simulink model "PassiveHydPTO"  (R2014a)
settings: Solver=ode23tb  StartTime=0.0  StopTime=param.stop  FixedStep=0.01  MaxStep=0.05  RelTol=1e-6
values from neighbouring files (symbols this model uses):
  alpha = 1    [passive_hydraulic_PTO.m]
  Amax = 0.001    [passive_hydraulic_PTO.m]
  Amin = 1e-8    (= 1e-08)    [passive_hydraulic_PTO.m]
  Ap = 2.35e-2    (= 0.0235)    [passive_hydraulic_PTO.m]
  Beta_e = 1.86e9    (= 1860000000)    [passive_hydraulic_PTO.m]
  bf = 0.05*bg    (= 0.118735)    [passive_hydraulic_PTO.m]
  bg = 2.3747    [passive_hydraulic_PTO.m]
  Cd = 0.61    [passive_hydraulic_PTO.m]
  D = 3.9789e-5    (= 3.9789e-05)    [passive_hydraulic_PTO.m]
  Dh = sqrt(4*Av/pi)    [passive_hydraulic_PTO.m]
  f = 1/period    (= 0.1)    [passive_hydraulic_PTO.m]
  J = 3.961    [passive_hydraulic_PTO.m]
  k1 = 200    [passive_hydraulic_PTO.m]
  k2 = atanh((Amin-(Amax-Amin)/2)*      2/(Amax - Amin))*1/(pMin-(pMax + pMin)/2)    [passive_hydraulic_PTO.m]
  omega_i = 0    [passive_hydraulic_PTO.m]
  pAeq = pCeq    (= 21333333.3333)    [passive_hydraulic_PTO.m]
  pAi = pAeq    (= 21333333.3333)    [passive_hydraulic_PTO.m]
  pAupper_limit = 32e6    (= 32000000)    [passive_hydraulic_PTO.m]
  pBeq = pCeq    (= 21333333.3333)    [passive_hydraulic_PTO.m]
  pBi = pBeq    (= 21333333.3333)    [passive_hydraulic_PTO.m]
  pBupper_limit = 32e6    (= 32000000)    [passive_hydraulic_PTO.m]
  pCprecharge = 0.9*pClower_limit    (= 19200000)    [passive_hydraulic_PTO.m]
  pDprecharge = 0.9*pDlower_limit    (= 9600000)    [passive_hydraulic_PTO.m]
  pMax = 1e6    (= 1000000)    [passive_hydraulic_PTO.m]
  pMin = 0.75e6    (= 750000)    [passive_hydraulic_PTO.m]
  rho = 850    [passive_hydraulic_PTO.m]
  Rt = 10    [passive_hydraulic_PTO.m]
  v = 5.5e-5    (= 5.5e-05)    [passive_hydraulic_PTO.m]
  VC0 = 7.5    [passive_hydraulic_PTO.m]
  VCeq = VC0*(1-(pCprecharge/pCeq)^(1/1.4))    (= 0.543715404282)    [passive_hydraulic_PTO.m]
  VD0 = 3    [passive_hydraulic_PTO.m]
  VDeq = VDmax    (= 1.30403881906)    [passive_hydraulic_PTO.m]
  Vo = Ap*5    (= 0.1175)    [passive_hydraulic_PTO.m]
undefined symbols (not defined in the file or in its folder): magnitude
settings Model: Creator=sor  LastModifiedBy=sor

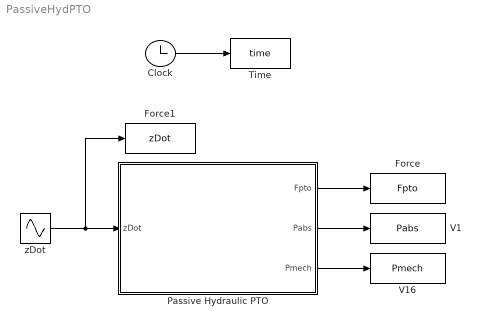
== system PassiveHydPTO ==
  Clock : Clock
  Force : ToWorkspace  VariableName=Fpto  SampleTime=-1
  Force1 : ToWorkspace  VariableName=zDot  SampleTime=-1
  "Passive Hydraulic PTO " : Subsystem
  Time : ToWorkspace  VariableName=time  SampleTime=-1
  V1 : ToWorkspace  VariableName=Pabs  SampleTime=-1
  V16 : ToWorkspace  VariableName=Pmech  SampleTime=-1
  zDot : Sin  Amplitude=0.8  Frequency=2*pi*f  SampleTime=0
  wires:
  "Passive Hydraulic PTO "/1(Fpto) -> Force/1
  Clock/1 -> Time/1
  "Passive Hydraulic PTO "/2(Pabs) -> V1/1
  zDot/1 -> "Passive Hydraulic PTO "/1(zDot), Force1/1
  "Passive Hydraulic PTO "/3(Pmech) -> V16/1

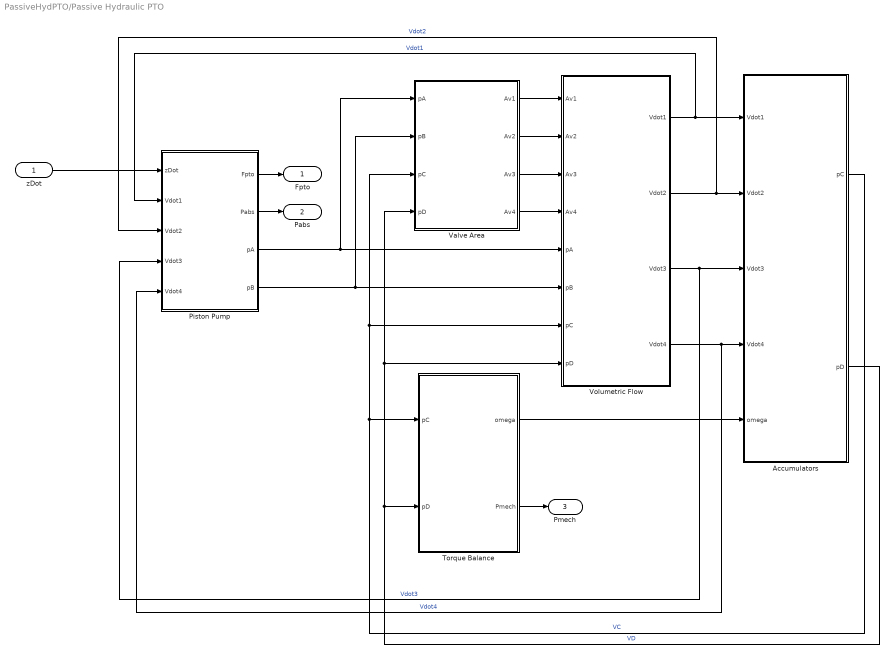
== system PassiveHydPTO/Passive Hydraulic PTO  ==
  zDot : Inport
  Accumulators : Subsystem
  "Piston Pump " : Subsystem
  Torque Balance : Subsystem
  Valve Area : Subsystem
  Volumetric Flow : Subsystem
  Fpto : Outport
  Pabs : Outport  Port=2
  Pmech : Outport  Port=3
  wires:
  zDot/1 -> "Piston Pump "/1(zDot)
  Valve Area/1(Av1) -> Volumetric Flow/1(Av1)
  Valve Area/2(Av2) -> Volumetric Flow/2(Av2)
  Valve Area/3(Av3) -> Volumetric Flow/3(Av3)
  Valve Area/4(Av4) -> Volumetric Flow/4(Av4)
  Volumetric Flow/1(Vdot1) -> Accumulators/1(Vdot1), "Piston Pump "/2(Vdot1)  "Vdot1"
  Volumetric Flow/2(Vdot2) -> "Piston Pump "/3(Vdot2), Accumulators/2(Vdot2)  "Vdot2"
  Volumetric Flow/3(Vdot3) -> Accumulators/3(Vdot3), "Piston Pump "/4(Vdot3)  "Vdot3"
  Volumetric Flow/4(Vdot4) -> "Piston Pump "/5(Vdot4), Accumulators/4(Vdot4)  "Vdot4"
  Accumulators/1(pC) -> Torque Balance/1(pC), Volumetric Flow/7(pC), Valve Area/3(pC)  "VC"
  Accumulators/2(pD) -> Torque Balance/2(pD), Volumetric Flow/8(pD), Valve Area/4(pD)  "VD"
  "Piston Pump "/3(pA) -> Volumetric Flow/5(pA), Valve Area/1(pA)
  "Piston Pump "/4(pB) -> Volumetric Flow/6(pB), Valve Area/2(pB)
  Torque Balance/1(omega) -> Accumulators/5(omega)
  Torque Balance/2(Pmech) -> Pmech/1
  "Piston Pump "/1(Fpto) -> Fpto/1
  "Piston Pump "/2(Pabs) -> Pabs/1

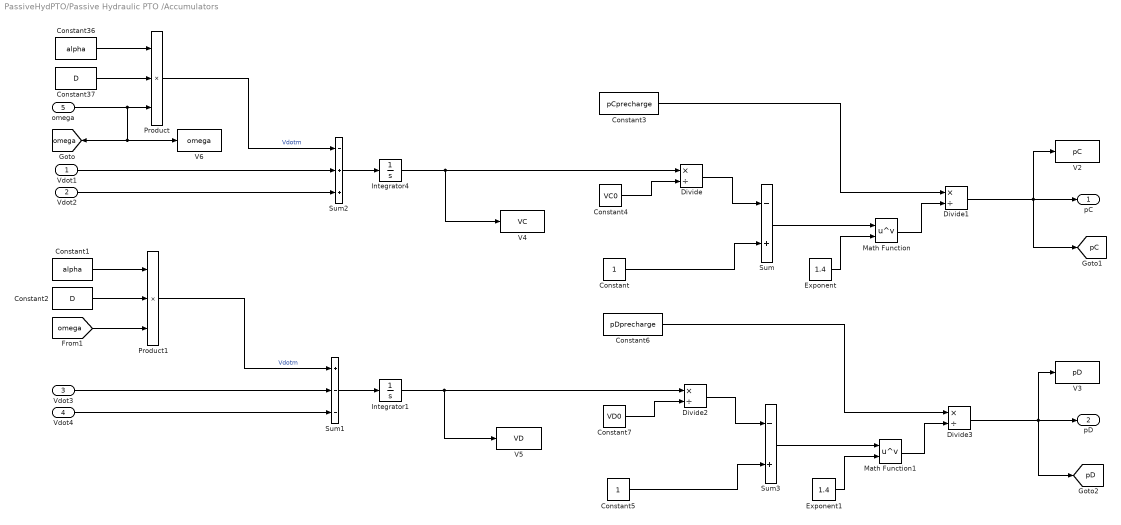
== system PassiveHydPTO/Passive Hydraulic PTO /Accumulators ==
  Vdot1 : Inport
  Vdot2 : Inport  Port=2
  Vdot3 : Inport  Port=3
  Vdot4 : Inport  Port=4
  omega : Inport  Port=5
  Constant : Constant
  Constant1 : Constant  Value=alpha
  Constant2 : Constant  Value=D
  Constant3 : Constant  Value=pCprecharge
  Constant36 : Constant  Value=alpha
  Constant37 : Constant  Value=D
  Constant4 : Constant  Value=VC0
  Constant5 : Constant
  Constant6 : Constant  Value=pDprecharge
  Constant7 : Constant  Value=VD0
  Divide{,1..3} (4 alike) : Product  Inputs=*/
  Exponent : Constant  Value=1.4
  Exponent1 : Constant  Value=1.4
  Integrator1 : Integrator  InitialCondition=VDeq
  Integrator4 : Integrator  InitialCondition=VCeq
  Math Function : Math  Operator=pow  SaturateOnIntegerOverflow=on
  Math Function1 : Math  Operator=pow  SaturateOnIntegerOverflow=on
  Product : Product  Inputs=3
  Product1 : Product  Inputs=3
  Sum : Sum  Inputs=-+
  Sum1 : Sum  Inputs=+--
  Sum2 : Sum  Inputs=-++
  Sum3 : Sum  Inputs=-+
  V2 : ToWorkspace  VariableName=pC  SampleTime=-1
  V3 : ToWorkspace  VariableName=pD  SampleTime=-1
  V4 : ToWorkspace  VariableName=VC  SampleTime=-1
  V5 : ToWorkspace  VariableName=VD  SampleTime=-1
  V6 : ToWorkspace  VariableName=omega  SampleTime=-1
  pC : Outport
  pD : Outport  Port=2
  tag scope: omega=global, pC=global, pD=global
  wires:
  Constant36/1 -> Product/1
  Constant37/1 -> Product/2
  omega/1 -> V6/1, [omega], Product/3
  Product/1 -> Sum2/1  "Vdotm"
  Vdot1/1 -> Sum2/2
  Vdot2/1 -> Sum2/3
  Sum2/1 -> Integrator4/1
  Constant1/1 -> Product1/1
  Constant2/1 -> Product1/2
  [omega] -> Product1/3
  Product1/1 -> Sum1/1  "Vdotm"
  Vdot3/1 -> Sum1/2
  Vdot4/1 -> Sum1/3
  Sum1/1 -> Integrator1/1
  Integrator4/1 -> Divide/1, V4/1
  Constant4/1 -> Divide/2
  Constant/1 -> Sum/2
  Divide/1 -> Sum/1
  Exponent/1 -> Math Function/2
  Sum/1 -> Math Function/1
  Math Function/1 -> Divide1/2
  Constant3/1 -> Divide1/1
  Integrator1/1 -> V5/1, Divide2/1
  Constant7/1 -> Divide2/2
  Constant5/1 -> Sum3/2
  Divide2/1 -> Sum3/1
  Exponent1/1 -> Math Function1/2
  Sum3/1 -> Math Function1/1
  Math Function1/1 -> Divide3/2
  Constant6/1 -> Divide3/1
  Divide1/1 -> [pC], V2/1, pC/1
  Divide3/1 -> [pD], V3/1, pD/1

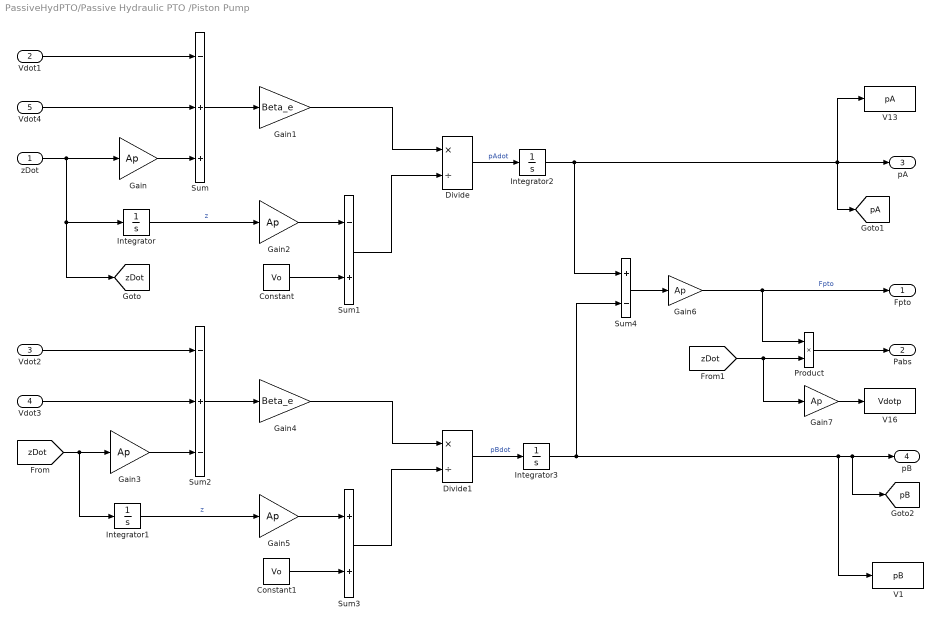
== system PassiveHydPTO/Passive Hydraulic PTO /Piston Pump  ==
  zDot : Inport
  Vdot1 : Inport  Port=2
  Vdot2 : Inport  Port=3
  Vdot3 : Inport  Port=4
  Vdot4 : Inport  Port=5
  Constant : Constant  Value=Vo
  Constant1 : Constant  Value=Vo
  Divide : Product  Inputs=*/
  Divide1 : Product  Inputs=*/
  Gain{,2..3,5..7} (6 alike) : Gain  Gain=Ap
  Gain1 : Gain  Gain=Beta_e
  Gain4 : Gain  Gain=Beta_e
  Integrator : Integrator
  Integrator1 : Integrator
  Integrator2 : Integrator  InitialCondition=pAi  UpperSaturationLimit=pAupper_limit  LowerSaturationLimit=pAeq
  Integrator3 : Integrator  InitialCondition=pBi  UpperSaturationLimit=pBupper_limit  LowerSaturationLimit=pBeq
  Product : Product
  Sum : Sum  Inputs=-++
  Sum1 : Sum  Inputs=-+
  Sum2 : Sum  Inputs=-+-
  Sum3 : Sum
  Sum4 : Sum  Inputs=+-
  V1 : ToWorkspace  VariableName=pB  SampleTime=-1
  V13 : ToWorkspace  VariableName=pA  SampleTime=-1
  V16 : ToWorkspace  VariableName=Vdotp  SampleTime=-1
  Fpto : Outport
  Pabs : Outport  Port=2
  pA : Outport  Port=3
  pB : Outport  Port=4
  tag scope: pA=global, pB=global, zDot=global
  wires:
  Gain/1 -> Sum/3
  Sum/1 -> Gain1/1
  zDot/1 -> Integrator/1, [zDot], Gain/1
  Integrator/1 -> Gain2/1  "z"
  Gain2/1 -> Sum1/1
  Constant/1 -> Sum1/2
  Gain1/1 -> Divide/1
  Sum1/1 -> Divide/2
  Vdot1/1 -> Sum/1
  Divide/1 -> Integrator2/1  "pAdot"
  Gain3/1 -> Sum2/3
  Sum2/1 -> Gain4/1
  [zDot] -> Integrator1/1, Gain3/1
  Integrator1/1 -> Gain5/1  "z"
  Gain5/1 -> Sum3/1
  Constant1/1 -> Sum3/2
  Gain4/1 -> Divide1/1
  Sum3/1 -> Divide1/2
  Divide1/1 -> Integrator3/1  "pBdot"
  Vdot4/1 -> Sum/2
  Vdot2/1 -> Sum2/1
  Vdot3/1 -> Sum2/2
  Sum4/1 -> Gain6/1
  Gain7/1 -> V16/1
  Gain6/1 -> Fpto/1, Product/1  "Fpto"
  [zDot] -> Gain7/1, Product/2
  Integrator3/1 -> V1/1, pB/1, [pB], Sum4/2
  Integrator2/1 -> pA/1, [pA], V13/1, Sum4/1
  Product/1 -> Pabs/1

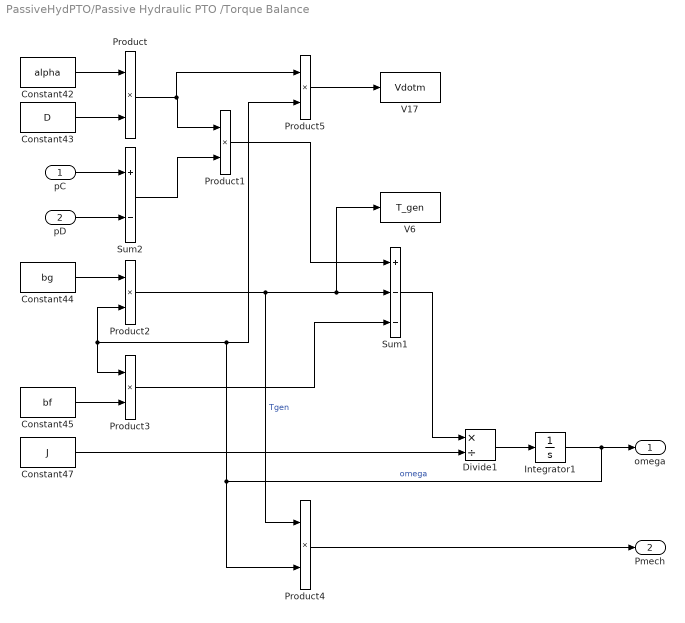
== system PassiveHydPTO/Passive Hydraulic PTO /Torque Balance ==
  pC : Inport
  pD : Inport  Port=2
  Constant42 : Constant  Value=alpha
  Constant43 : Constant  Value=D
  Constant44 : Constant  Value=bg
  Constant45 : Constant  Value=bf
  Constant47 : Constant  Value=J
  Divide1 : Product  Inputs=*/
  Integrator1 : Integrator  InitialCondition=omega_i
  Product{,1..5} (6 alike) : Product
  Sum1 : Sum  Inputs=+--
  Sum2 : Sum  Inputs=+-
  V17 : ToWorkspace  VariableName=Vdotm  SampleTime=-1
  V6 : ToWorkspace  VariableName=T_gen  SampleTime=-1
  omega : Outport
  Pmech : Outport  Port=2
  wires:
  Constant42/1 -> Product/1
  Constant43/1 -> Product/2
  pC/1 -> Sum2/1
  pD/1 -> Sum2/2
  Product/1 -> Product5/1, Product1/1
  Sum2/1 -> Product1/2
  Constant44/1 -> Product2/1
  Constant45/1 -> Product3/2
  Product1/1 -> Sum1/1
  Product2/1 -> Product4/1, V6/1, Sum1/2  "Tgen"
  Product3/1 -> Sum1/3
  Sum1/1 -> Divide1/1
  Constant47/1 -> Divide1/2
  Product4/1 -> Pmech/1
  Divide1/1 -> Integrator1/1
  Integrator1/1 -> omega/1, Product4/2, Product3/1, Product2/2, Product5/2  "omega"
  Product5/1 -> V17/1

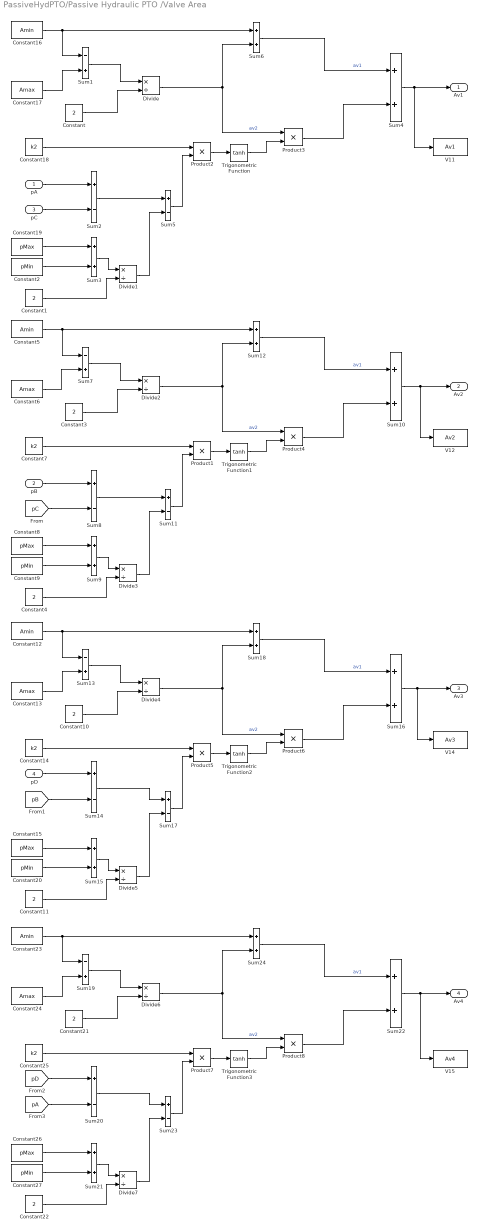
== system PassiveHydPTO/Passive Hydraulic PTO /Valve Area ==
  pA : Inport
  pB : Inport  Port=2
  pC : Inport  Port=3
  pD : Inport  Port=4
  Constant{,1,3..4,10..11,21..22} (8 alike) : Constant  Value=2
  Constant{5,12,16,23} (4 alike) : Constant  Value=Amin
  Constant{6,13,17,24} (4 alike) : Constant  Value=Amax
  Constant{7,14,18,25} (4 alike) : Constant  Value=k2
  Constant{8,15,19,26} (4 alike) : Constant  Value=pMax
  Constant{2,9,20,27} (4 alike) : Constant  Value=pMin
  Divide{,1..7} (8 alike) : Product  Inputs=*/
  Product{1..8} (8 alike) : Product
  Sum{1,7,13,19} (4 alike) : Sum  Inputs=-+
  Sum{3..4,6,9..10,12,15..16,18,21..22,24} (12 alike) : Sum
  Sum{2,5,8,11,14,17,20,23} (8 alike) : Sum  Inputs=+-
  Trigonometric Function{,1..3} (4 alike) : Trigonometry  Operator=tanh
  V11 : ToWorkspace  VariableName=Av1  SampleTime=-1
  V12 : ToWorkspace  VariableName=Av2  SampleTime=-1
  V14 : ToWorkspace  VariableName=Av3  SampleTime=-1
  V15 : ToWorkspace  VariableName=Av4  SampleTime=-1
  Av1 : Outport
  Av2 : Outport  Port=2
  Av3 : Outport  Port=3
  Av4 : Outport  Port=4
  wires:
  Constant16/1 -> Sum6/1, Sum1/1
  Constant17/1 -> Sum1/2
  Sum1/1 -> Divide/1
  Constant/1 -> Divide/2
  Product2/1 -> Trigonometric Function/1
  Trigonometric Function/1 -> Product3/2
  Product3/1 -> Sum4/2
  pA/1 -> Sum2/1
  Constant19/1 -> Sum3/1
  Constant2/1 -> Sum3/2
  Sum3/1 -> Divide1/1
  Constant1/1 -> Divide1/2
  Divide/1 -> Sum6/2, Product3/1  "av2"
  Sum4/1 -> V11/1, Av1/1
  Sum2/1 -> Sum5/1
  Divide1/1 -> Sum5/2
  Constant18/1 -> Product2/1
  Sum5/1 -> Product2/2
  Sum6/1 -> Sum4/1  "av1"
  Constant5/1 -> Sum12/1, Sum7/1
  Constant6/1 -> Sum7/2
  Sum7/1 -> Divide2/1
  Constant3/1 -> Divide2/2
  Product1/1 -> Trigonometric Function1/1
  Trigonometric Function1/1 -> Product4/2
  Product4/1 -> Sum10/2
  Constant8/1 -> Sum9/1
  Constant9/1 -> Sum9/2
  Sum9/1 -> Divide3/1
  Constant4/1 -> Divide3/2
  Divide2/1 -> Sum12/2, Product4/1  "av2"
  Sum10/1 -> V12/1, Av2/1
  Sum8/1 -> Sum11/1
  Divide3/1 -> Sum11/2
  Constant7/1 -> Product1/1
  Sum11/1 -> Product1/2
  Sum12/1 -> Sum10/1  "av1"
  Constant12/1 -> Sum18/1, Sum13/1
  Constant13/1 -> Sum13/2
  Sum13/1 -> Divide4/1
  Constant10/1 -> Divide4/2
  Product5/1 -> Trigonometric Function2/1
  Trigonometric Function2/1 -> Product6/2
  Product6/1 -> Sum16/2
  Constant15/1 -> Sum15/1
  Constant20/1 -> Sum15/2
  Sum15/1 -> Divide5/1
  Constant11/1 -> Divide5/2
  Divide4/1 -> Sum18/2, Product6/1  "av2"
  Sum14/1 -> Sum17/1
  Divide5/1 -> Sum17/2
  Constant14/1 -> Product5/1
  Sum17/1 -> Product5/2
  Sum18/1 -> Sum16/1  "av1"
  Constant23/1 -> Sum24/1, Sum19/1
  Constant24/1 -> Sum19/2
  Sum19/1 -> Divide6/1
  Constant21/1 -> Divide6/2
  Product7/1 -> Trigonometric Function3/1
  Trigonometric Function3/1 -> Product8/2
  Product8/1 -> Sum22/2
  Constant26/1 -> Sum21/1
  Constant27/1 -> Sum21/2
  Sum21/1 -> Divide7/1
  Constant22/1 -> Divide7/2
  Divide6/1 -> Sum24/2, Product8/1  "av2"
  Sum22/1 -> V15/1, Av4/1
  Sum20/1 -> Sum23/1
  Divide7/1 -> Sum23/2
  Constant25/1 -> Product7/1
  Sum23/1 -> Product7/2
  Sum24/1 -> Sum22/1  "av1"
  pC/1 -> Sum2/2
  pB/1 -> Sum8/1
  [pC] -> Sum8/2
  pD/1 -> Sum14/1
  [pB] -> Sum14/2
  [pD] -> Sum20/1
  [pA] -> Sum20/2
  Sum16/1 -> V14/1, Av3/1

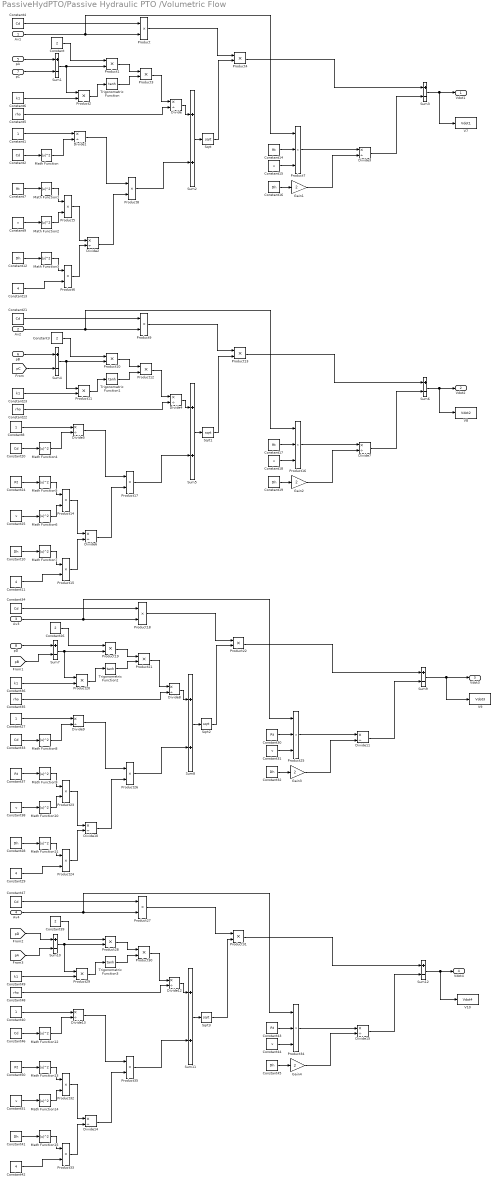
== system PassiveHydPTO/Passive Hydraulic PTO /Volumetric Flow ==
  Av1 : Inport
  Av2 : Inport  Port=2
  Av3 : Inport  Port=3
  Av4 : Inport  Port=4
  pA : Inport  Port=5
  pB : Inport  Port=6
  pC : Inport  Port=7
  pD : Inport  Port=8
  Constant{,3,26,39} (4 alike) : Constant  Value=2
  Constant{1,8,27,40} (4 alike) : Constant
  Constant{10,12,16,19,28,32,41,45} (8 alike) : Constant  Value=Dh
  Constant{11,13,29,42} (4 alike) : Constant  Value=4
  Constant{7,14,17,24,30,37,43,50} (8 alike) : Constant  Value=Rt
  Constant{9,15,18,25,31,38,44,51} (8 alike) : Constant  Value=v
  Constant{2,4,20..21,33..34,46..47} (8 alike) : Constant  Value=Cd
  Constant{5,22,35,48} (4 alike) : Constant  Value=rho
  Constant{6,23,36,49} (4 alike) : Constant  Value=k1
  Divide{,1..15} (16 alike) : Product  Inputs=*/
  Gain{1..4} (4 alike) : Gain  Gain=2
  Math Function{,1..15} (16 alike) : Math  Operator=magnitude^2  SaturateOnIntegerOverflow=on
  Product{,1..6,8..15,17..24,26..33,35} (32 alike) : Product
  Product{7,16,25,34} (4 alike) : Product  Inputs=3
  Sqrt{,1..3} (4 alike) : Sqrt  SaturateOnIntegerOverflow=on
  Sum{1,3..4,6..7,9..10,12} (8 alike) : Sum  Inputs=+-
  Sum{2,5,8,11} (4 alike) : Sum
  Trigonometric Function{,1..3} (4 alike) : Trigonometry  Operator=tanh
  V10 : ToWorkspace  VariableName=Vdot4  SampleTime=-1
  V7 : ToWorkspace  VariableName=Vdot1  SampleTime=-1
  V8 : ToWorkspace  VariableName=Vdot2  SampleTime=-1
  V9 : ToWorkspace  VariableName=Vdot3  SampleTime=-1
  Vdot1 : Outport
  Vdot2 : Outport  Port=2
  Vdot3 : Outport  Port=3
  Vdot4 : Outport  Port=4
  wires:
  Constant4/1 -> Product/1
  Av1/1 -> Product/2, Product7/1
  Sum1/1 -> Product2/1, Product1/2
  Constant/1 -> Product1/1
  Constant6/1 -> Product2/2
  Product2/1 -> Trigonometric Function/1
  Product1/1 -> Product3/1
  Trigonometric Function/1 -> Product3/2
  Sqrt/1 -> Product4/2
  Product/1 -> Product4/1
  Constant5/1 -> Divide/2
  Product3/1 -> Divide/1
  Divide/1 -> Sum2/1
  Sum2/1 -> Sqrt/1
  Product4/1 -> Sum3/1
  Constant14/1 -> Product7/2
  Constant15/1 -> Product7/3
  Product7/1 -> Divide3/1
  Constant16/1 -> Gain1/1
  Gain1/1 -> Divide3/2
  Divide3/1 -> Sum3/2
  Product8/1 -> Sum2/2
  Constant1/1 -> Divide1/1
  Constant2/1 -> Math Function/1
  Math Function/1 -> Divide1/2
  Constant7/1 -> Math Function1/1
  Constant9/1 -> Math Function2/1
  Math Function1/1 -> Product5/1
  Math Function2/1 -> Product5/2
  Constant12/1 -> Math Function3/1
  Math Function3/1 -> Product6/1
  Constant13/1 -> Product6/2
  Product5/1 -> Divide2/1
  Product6/1 -> Divide2/2
  Divide1/1 -> Product8/1
  Divide2/1 -> Product8/2
  Constant21/1 -> Product9/1
  Av2/1 -> Product9/2, Product16/1
  Sum4/1 -> Product11/1, Product10/2
  Constant3/1 -> Product10/1
  Constant23/1 -> Product11/2
  Product11/1 -> Trigonometric Function1/1
  Product10/1 -> Product12/1
  Trigonometric Function1/1 -> Product12/2
  Sqrt1/1 -> Product13/2
  Product9/1 -> Product13/1
  Constant22/1 -> Divide4/2
  Product12/1 -> Divide4/1
  Product13/1 -> Sum6/1
  Constant17/1 -> Product16/2
  Constant18/1 -> Product16/3
  Product16/1 -> Divide7/1
  Constant19/1 -> Gain2/1
  Gain2/1 -> Divide7/2
  Divide7/1 -> Sum6/2
  Sum6/1 -> V8/1, Vdot2/1
  Sum5/1 -> Sqrt1/1
  Product17/1 -> Sum5/2
  Divide4/1 -> Sum5/1
  Constant8/1 -> Divide5/1
  Constant20/1 -> Math Function4/1
  Math Function4/1 -> Divide5/2
  Constant24/1 -> Math Function5/1
  Constant25/1 -> Math Function6/1
  Math Function5/1 -> Product14/1
  Math Function6/1 -> Product14/2
  Constant10/1 -> Math Function7/1
  Math Function7/1 -> Product15/1
  Constant11/1 -> Product15/2
  Product14/1 -> Divide6/1
  Product15/1 -> Divide6/2
  Divide5/1 -> Product17/1
  Divide6/1 -> Product17/2
  Constant34/1 -> Product18/1
  Av3/1 -> Product18/2, Product25/1
  pD/1 -> Sum7/1
  [pB] -> Sum7/2
  Sum7/1 -> Product20/1, Product19/2
  Constant26/1 -> Product19/1
  Constant36/1 -> Product20/2
  Product20/1 -> Trigonometric Function2/1
  Product19/1 -> Product21/1
  Trigonometric Function2/1 -> Product21/2
  Sqrt2/1 -> Product22/2
  Product18/1 -> Product22/1
  Constant35/1 -> Divide8/2
  Product21/1 -> Divide8/1
  Product22/1 -> Sum9/1
  Constant30/1 -> Product25/2
  Constant31/1 -> Product25/3
  Product25/1 -> Divide11/1
  Constant32/1 -> Gain3/1
  Gain3/1 -> Divide11/2
  Divide11/1 -> Sum9/2
  Sum8/1 -> Sqrt2/1
  Product26/1 -> Sum8/2
  Divide8/1 -> Sum8/1
  Constant27/1 -> Divide9/1
  Constant33/1 -> Math Function8/1
  Math Function8/1 -> Divide9/2
  Constant37/1 -> Math Function9/1
  Constant38/1 -> Math Function10/1
  Math Function9/1 -> Product23/1
  Math Function10/1 -> Product23/2
  Constant28/1 -> Math Function11/1
  Math Function11/1 -> Product24/1
  Constant29/1 -> Product24/2
  Product23/1 -> Divide10/1
  Product24/1 -> Divide10/2
  Divide9/1 -> Product26/1
  Divide10/1 -> Product26/2
  Sum9/1 -> V9/1, Vdot3/1
  Constant47/1 -> Product27/1
  Av4/1 -> Product27/2, Product34/1
  [pD] -> Sum10/1
  [pA] -> Sum10/2
  Sum10/1 -> Product29/1, Product28/2
  Constant39/1 -> Product28/1
  Constant49/1 -> Product29/2
  Product29/1 -> Trigonometric Function3/1
  Product28/1 -> Product30/1
  Trigonometric Function3/1 -> Product30/2
  Product27/1 -> Product31/1
  Constant48/1 -> Divide12/2
  Product30/1 -> Divide12/1
  Constant40/1 -> Divide13/1
  Constant46/1 -> Math Function12/1
  Math Function12/1 -> Divide13/2
  Constant50/1 -> Math Function13/1
  Constant51/1 -> Math Function14/1
  Math Function13/1 -> Product32/1
  Math Function14/1 -> Product32/2
  Constant41/1 -> Math Function15/1
  Math Function15/1 -> Product33/1
  Constant42/1 -> Product33/2
  Product32/1 -> Divide14/1
  Product33/1 -> Divide14/2
  Product31/1 -> Sum12/1
  Constant43/1 -> Product34/2
  Constant44/1 -> Product34/3
  Product34/1 -> Divide15/1
  Constant45/1 -> Gain4/1
  Gain4/1 -> Divide15/2
  Divide15/1 -> Sum12/2
  Sum11/1 -> Sqrt3/1
  Divide13/1 -> Product35/1
  Divide14/1 -> Product35/2
  Product35/1 -> Sum11/2
  Divide12/1 -> Sum11/1
  Sqrt3/1 -> Product31/2
  Sum12/1 -> V10/1, Vdot4/1
  pA/1 -> Sum1/1
  pC/1 -> Sum1/2
  pB/1 -> Sum4/1
  [pC] -> Sum4/2
  Sum3/1 -> V7/1, Vdot1/1
